simulink model "closedloop_statefeedback_ref"  (R2015a)
settings: Solver=ode45  StartTime=0.0  StopTime=60  FixedStep=1e-3  MaxStep=1e-2  RelTol=1e-3
undefined symbols (not defined in the file): A, B, C, K1, N1
libraries: simulink_extras x1
settings Model: Creator=henrik  LastModifiedBy=hg35a
settings DataIOCC: SignalLoggingSaveFormat=ModelDataLogs  SignalLoggingName=sigsOut
settings OptimizationCC: ExpressionDepthLimit=2147483647  InitFltsAndDblsToZero=on
settings DebuggingCC: SaveWithParameterizedLinksMsg=none  UnderspecifiedInitializationDetection=Classic  MergeDetectMultiDrivingBlocksExec=none  SignalResolutionControl=TryResolveAllWithWarning  MultiTaskDSMMsg=warning  MultiTaskCondExecSysMsg=none  FcnCallInpInsideContextMsg=UseLocalSettings  StateNameClashWarn=warning
settings HardwareCC: TargetUnknown=on
settings GRTTargetCC: TargetFcnLib=ansi_tfl_tmw.mat  ModelReferenceCompliant=off  CombineOutputUpdateFcns=off  MatFileLogging=off  GRTInterface=on

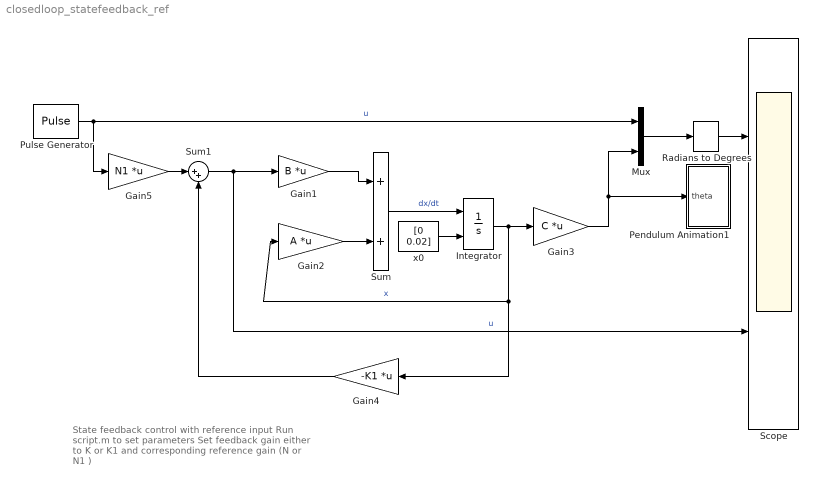
== system closedloop_statefeedback_ref ==
  note: State feedback control with reference input
      | Run script.m to set parameters
      | Set feedback gain either to K or K1
      | and corresponding reference gain (N or N1 )
  Gain1 : Gain  Gain=B  Multiplication=Matrix(K*u)  SaturateOnIntegerOverflow=on  OutDataTypeStr=Inherit: Same as input  ParamDataTypeStr=Inherit: Same as input
  Gain2 : Gain  Gain=A  Multiplication=Matrix(K*u)  SaturateOnIntegerOverflow=on  OutDataTypeStr=Inherit: Same as input  ParamDataTypeStr=Inherit: Same as input
  Gain3 : Gain  Gain=C  Multiplication=Matrix(K*u)  SaturateOnIntegerOverflow=on  OutDataTypeStr=Inherit: Same as input  ParamDataTypeStr=Inherit: Same as input
  Gain4 : Gain  Gain=-K1  Multiplication=Matrix(K*u)  SaturateOnIntegerOverflow=on  OutDataTypeStr=Inherit: Same as input  ParamDataTypeStr=Inherit: Same as input
  Gain5 : Gain  Gain=N1  Multiplication=Matrix(K*u)  SaturateOnIntegerOverflow=on  OutDataTypeStr=Inherit: Same as input  ParamDataTypeStr=Inherit: Same as input
  Integrator : Integrator  InitialConditionSource=external
  Mux : Mux  Inputs=2
  Pendulum Animation1 : Subsystem
  Pulse Generator : DiscretePulseGenerator  PulseType=Time based  Amplitude=10*pi/180  Period=10  PulseWidth=50
      settings: AttributesFormatString=Amplitude=%<Amplitude>
  Radians to Degrees : simulink_extras/Transformations/Radians to Degrees
  Scope : Scope  NumInputPorts=2
      settings: YMin=-5~-25  YMax=12.5~15
  Sum : Sum  SaturateOnIntegerOverflow=on  InputSameDT=on  OutDataTypeStr=Inherit: Same as first input
  Sum1 : Sum  Inputs=|++
  x0 : Constant  Value=[0 0.02]
  wires:
  Gain1/1 -> Sum/1
  Gain2/1 -> Sum/2
  Sum/1 -> Integrator/1  "dx/dt"
  Integrator/1 -> Gain3/1, Gain2/1, Gain4/1  "x"
  Pulse Generator/1 -> Mux/1, Gain5/1  "u"
  Mux/1 -> Radians to Degrees/1
  Gain3/1 -> Mux/2, Pendulum Animation1/1(theta)
  Sum1/1 -> Gain1/1, Scope/2  "u"
  Gain5/1 -> Sum1/1
  Radians to Degrees/1 -> Scope/1
  Gain4/1 -> Sum1/2
  x0/1 -> Integrator/2

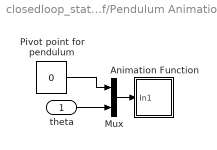
== system closedloop_statefeedback_ref/Pendulum Animation1 ==
  theta : Inport
  Animation Function : Subsystem  mask(Animation Block){ts=0.01}
      mask prompts: ts "Sample time:"
      mask Display: plot([.1,.9],[.9,.9],[.5,.2],[.9,.25],[.475,.475,.525,.525,.475],[.875,.925,.925,.875,.875])
  Mux : Mux  Inputs=2
  Pivot point for pendulum : Constant  Value=0
  wires:
  theta/1 -> Mux/2
  Pivot point for pendulum/1 -> Mux/1
  Mux/1 -> Animation Function/1(In1)

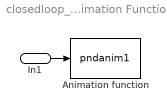
== system closedloop_statefeedback_ref/Pendulum Animation1/Animation Function ==
  In1 : Inport
  Animation function : S-Function  FunctionName=pndanim1  Parameters=ts
      settings: DeleteFcn=if ~isempty(findobj('type','figure','name','simppend Animation'));close('simppend Animation'); end;
  wires:
  In1/1 -> Animation function/1
